simulink model "mission_planner_incremental_test"  (R2016b)
settings: Solver=VariableStepAuto  StartTime=0.0  StopTime=inf  RelTol=1e-3
model workspace (MAT data in the model file):
  SL_ROS_VariableLengthArrays_MaxSizes.CommonInfo.ArrayTruncateAction = 'EmitWarning'
  SL_ROS_VariableLengthArrays_MaxSizes.MsgTypeMap = containers.Map
  SL_ROS_VariableLengthArrays_MaxSizes.MsgTypeMap.serialization.keys = {'nav_msgs/OccupancyGrid'}
  SL_ROS_VariableLengthArrays_MaxSizes.MsgTypeMap.serialization.values{1}.PropertyName = 'Data'
  SL_ROS_VariableLengthArrays_MaxSizes.MsgTypeMap.serialization.values{1}.DataType = 'int8'
  SL_ROS_VariableLengthArrays_MaxSizes.MsgTypeMap.serialization.values{1}.MaxLength = 1048576
  SL_ROS_VariableLengthArrays_MaxSizes.MsgTypeMap.serialization.uniformity = 0
  SL_ROS_VariableLengthArrays_MaxSizes.MsgTypeMap.serialization.keyType = 'char'
  SL_ROS_VariableLengthArrays_MaxSizes.MsgTypeMap.serialization.valueType = 'any'
undefined symbols (not defined in the file): X, Y
libraries: robotlib x4, simulink x1
settings Model: Creator=aaron  LastModifiedBy=aaron

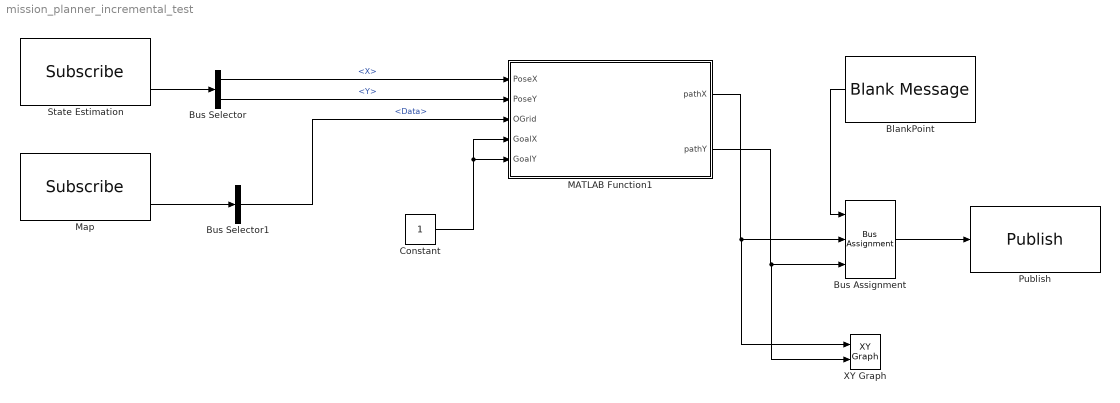
== system mission_planner_incremental_test ==
  BlankPoint : robotlib/Blank Message  SourceLibraryInfo=This block requires Robotics System Toolbox  messageType=geometry_msgs/Point  SampleTime=inf
  Bus Assignment : BusAssignment  AssignedSignals=X,Y
  Bus Selector : BusSelector  OutputSignals=Pose.Position.X,Pose.Position.Y
  Bus Selector1 : BusSelector  OutputSignals=Data
  Constant : Constant
  MATLAB Function1 : MATLAB Function  TreatAsAtomicUnit=on
  Map : robotlib/Subscribe  SourceLibraryInfo=This block requires Robotics System Toolbox  topicSource=Specify your own  topic=/map  messageType=nav_msgs/OccupancyGrid  sampleTime=-1  messageQueueLength=1
  Publish : robotlib/Publish  SourceLibraryInfo=This block requires Robotics System Toolbox  topicSource=Specify your own  topic=/GoTo  messageType=geometry_msgs/Point  messageQueueLength=1
  State Estimation : robotlib/Subscribe  SourceLibraryInfo=This block requires Robotics System Toolbox  topicSource=Specify your own  topic=/slam_out_pose  messageType=geometry_msgs/PoseStamped  sampleTime=-1  messageQueueLength=1
  XY Graph : simulink/Sinks/XY Graph  xmin=-1  xmax=1  ymin=-1  ymax=1  st=-1
  wires:
  BlankPoint/1 -> Bus Assignment/1
  Bus Assignment/1 -> Publish/1
  State Estimation/2 -> Bus Selector/1
  Bus Selector/1 -> MATLAB Function1/1(PoseX)  "<X>"
  Bus Selector/2 -> MATLAB Function1/2(PoseY)  "<Y>"
  MATLAB Function1/1(pathX) -> XY Graph/1, Bus Assignment/2
  MATLAB Function1/2(pathY) -> XY Graph/2, Bus Assignment/3
  Constant/1 -> MATLAB Function1/5(GoalY), MATLAB Function1/4(GoalX)
  Map/2 -> Bus Selector1/1
  Bus Selector1/1 -> MATLAB Function1/3(OGrid)  "<Data>"

== matlab function mission_planner_incremental_test/MATLAB Function1 ==
  data: PoseX input; PoseY input; OGrid input; GoalX input; GoalY input; pathX output; pathY output
function [pathX, pathY] = fcn(PoseX, PoseY, OGrid, GoalX, GoalY)
%#codegen

% Interpret data
    currPos = [PoseX, PoseY];


% Create a D* Object using the map
    [map, currPos] = convO2M(OGrid, currPos)
    goal = [GoalX, GoalY];
    start= currPos;
    MapConversionFinished=1
    ds = Dstar(map);
    DSMapFinished=1
    ds.plan(goal);

    spath = ds.path(start);

    spath


    % Publish path information
    pathX = spath(:, 1);
    pathY = spath(:, 2);
end
